simulink library "RFFTLib"  (R2022b)
settings: Solver=VariableStepAuto  StartTime=0.0  StopTime=10.0  RelTol=1e-3
settings Model: Creator=ud1041536  LastModifiedBy=kl13806
settings SolverCC: AlgebraicLoopSolver=TrustRegion
settings DebuggingCC: UnconnectedInputMsg=warning  UnconnectedOutputMsg=warning  UnconnectedLineMsg=warning  SFMachineParentedDataDiag=warning  ArithmeticOperatorsInVariantConditions=warning
settings ModelReferenceCC: EnableRefExpFcnMdlSchedulingChecks=on
settings SFSimCC: CustomCodeUndefinedFunction=UseInterfaceOnly
settings RTWCC: DLArmComputeVersion=19.05

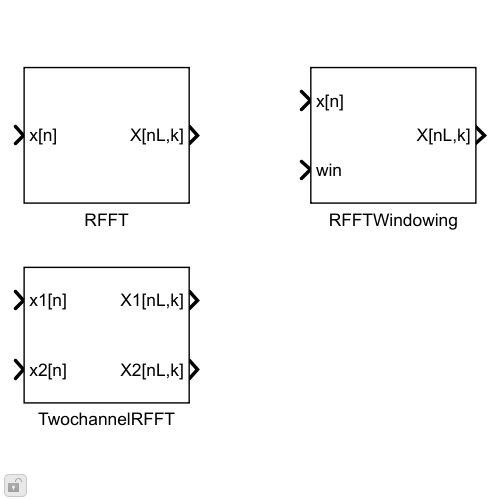
[thumbnail: Simulink's stored preview of the top-level diagram]
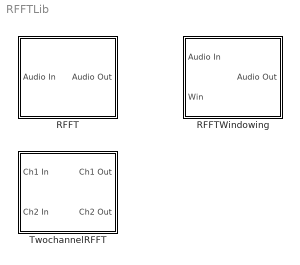
== system RFFTLib ==
  RFFT : Subsystem  mask(Real FFT){variantSelect=Core, fftSize=256, bufferAlias=default}
      mask prompts: variantSelect "Implementation:"; fftSize "FFT size"; bufferAlias "Alias (must be unique across all instances in model)"
      mask help:
      | This block computes the Fourier Transform using an optimized FFT for real inputs. It only supports even number of channels, and 128-point or 256-point FFT.
      |
      | 2 current implementation types are:
      | (i) Core
      | (ii) Generic
      mask init:
      | RfftMaskInit(gcbh, fftSize, bufferAlias, variantSelect)
      mask TypeOptions variantSelect: Core | Generic
      mask Display:
      | port_label('input',1,'x[n]')
      | port_label('output',1,'X[nL,k]')
  RFFTWindowing : Subsystem  mask(Real FFT with In-place Windowing){variantSelect=Core, fftSize=256, bufferAlias=default}
      mask prompts: variantSelect "Implementation:"; fftSize "FFT size"; bufferAlias "Alias (must be unique across all instances in model)"
      mask help:
      | This block performs in-place windowing followed by an optimized FFT computation for real inputs. It only supports even number of channels, and 128-point or 256-point FFT.
      |
      | 2 current implementation types are:
      | (i) Core
      | (ii) Generic
      mask init:
      | RfftMaskInit(gcbh, fftSize, bufferAlias, variantSelect)
      mask TypeOptions variantSelect: Core | Generic
      mask Display:
      | port_label('input',1,'x[n]')
      | port_label('input',2,'win')
      | port_label('output',1,'X[nL,k]')
  TwochannelRFFT : Subsystem  mask(In-place Real FFT){variantSelect=Core, fftSize=256, bufferAlias=default}
      mask prompts: variantSelect "Implementation:"; fftSize "FFT size"; bufferAlias "Alias (must be unique across all instances in model)"
      mask help:
      | This block computes the Fourier Transform using an optimized FFT for real 2-channel input. It only supports 128-point or 256-point FFT.
      |
      | 2 current implementation types are:
      | (i) Core
      | (ii) Generic
      |
      | The inputs MUST be configured correctly for the block to work. Please see 'Help' for more information.
      mask init:
      | Rfft2chanMaskInit(gcbh, fftSize, bufferAlias, variantSelect)
      mask Help:
      | <b>How to configure inputs:</b>
      | 
      | - Signal object class: <b>Blocklib.Signal</b>
      | - Storage class: <b>FFT Buffer</b>
      | - Memory section: <b>FFTMemL1DmWordAlign[fftSize]</b>for the first input signal, and <b>FFTMemL1PmWordAlign[fftSize]</b> for the second
      | 
      | 
      | <b>Why this configuration is needed: </b>
      | 
      | Since the Core implementation makes use of the processor SIMD's capability, the function imposes the following memory restrictions:
      | 1. All buffers (inputs, temp, twiddle) must be allocated in internal memory and not on stack.
      | 2. The inputs must be aligned on an address boundary that is a multiple of the FFT size.
      | 3. The first channel is allocated in a separate memory block from the second channel, i.e. the first one in Data memory and the second in Program memory.
      mask TypeOptions variantSelect: Core | Generic
      mask Display:
      | port_label('input',1,'x1[n]')
      | port_label('input',2,'x2[n]')
      | port_label('output',1,'X1[nL,k]')
      | port_label('output',2,'X2[nL,k]')

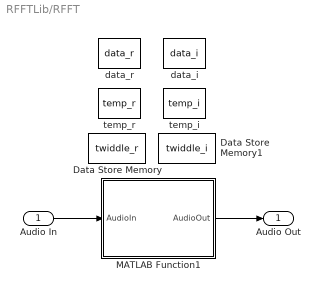
== system RFFTLib/RFFT ==
  Audio In : Inport
  Data Store Memory : DataStoreMemory  DataStoreName=twiddle_r  ReadBeforeWriteMsg=warning  WriteAfterWriteMsg=warning  WriteAfterReadMsg=warning  ShowAdditionalParam=off  OutDataTypeStr=uint32
  Data Store Memory1 : DataStoreMemory  DataStoreName=twiddle_i  ReadBeforeWriteMsg=warning  WriteAfterWriteMsg=warning  WriteAfterReadMsg=warning  ShowAdditionalParam=off  OutDataTypeStr=uint32
  MATLAB Function1 : MATLAB Function  TreatAsAtomicUnit=on
  data_i : DataStoreMemory  DataStoreName=data_i  ReadBeforeWriteMsg=warning  WriteAfterWriteMsg=warning  WriteAfterReadMsg=warning  InitialValue=zeros(fftSize,1)  EmbeddedSignalClassName=Blocklib.Signal  ShowAdditionalParam=off  OutDataTypeStr=single
  data_r : DataStoreMemory  DataStoreName=data_r  ReadBeforeWriteMsg=warning  WriteAfterWriteMsg=warning  WriteAfterReadMsg=warning  InitialValue=zeros(fftSize,1)  EmbeddedSignalClassName=Blocklib.Signal  ShowAdditionalParam=off  OutDataTypeStr=single
  temp_i : DataStoreMemory  DataStoreName=temp_i  ReadBeforeWriteMsg=warning  WriteAfterWriteMsg=warning  WriteAfterReadMsg=warning  InitialValue=zeros(fftSize,1)  EmbeddedSignalClassName=Blocklib.Signal  ShowAdditionalParam=off  OutDataTypeStr=single
  temp_r : DataStoreMemory  DataStoreName=temp_r  ReadBeforeWriteMsg=warning  WriteAfterWriteMsg=warning  WriteAfterReadMsg=warning  InitialValue=zeros(fftSize,1)  EmbeddedSignalClassName=Blocklib.Signal  ShowAdditionalParam=off  OutDataTypeStr=single
  Audio Out : Outport  VectorParamsAs1DForOutWhenUnconnected=off
  wires:
  MATLAB Function1/1(AudioOut) -> Audio Out/1
  Audio In/1 -> MATLAB Function1/1(AudioIn)

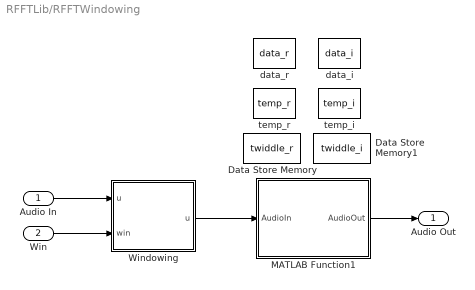
== system RFFTLib/RFFTWindowing ==
  Audio In : Inport
  Win : Inport  Port=2
  Data Store Memory : DataStoreMemory  DataStoreName=twiddle_r  ReadBeforeWriteMsg=warning  WriteAfterWriteMsg=warning  WriteAfterReadMsg=warning  ShowAdditionalParam=off  OutDataTypeStr=uint32
  Data Store Memory1 : DataStoreMemory  DataStoreName=twiddle_i  ReadBeforeWriteMsg=warning  WriteAfterWriteMsg=warning  WriteAfterReadMsg=warning  ShowAdditionalParam=off  OutDataTypeStr=uint32
  MATLAB Function1 : MATLAB Function  TreatAsAtomicUnit=on
  Windowing : MATLAB Function  TreatAsAtomicUnit=on
  data_i : DataStoreMemory  DataStoreName=data_i  ReadBeforeWriteMsg=warning  WriteAfterWriteMsg=warning  WriteAfterReadMsg=warning  InitialValue=zeros(fftSize,1)  EmbeddedSignalClassName=Blocklib.Signal  ShowAdditionalParam=off  OutDataTypeStr=single
  data_r : DataStoreMemory  DataStoreName=data_r  ReadBeforeWriteMsg=warning  WriteAfterWriteMsg=warning  WriteAfterReadMsg=warning  InitialValue=zeros(fftSize,1)  EmbeddedSignalClassName=Blocklib.Signal  ShowAdditionalParam=off  OutDataTypeStr=single
  temp_i : DataStoreMemory  DataStoreName=temp_i  ReadBeforeWriteMsg=warning  WriteAfterWriteMsg=warning  WriteAfterReadMsg=warning  InitialValue=zeros(fftSize,1)  EmbeddedSignalClassName=Blocklib.Signal  ShowAdditionalParam=off  OutDataTypeStr=single
  temp_r : DataStoreMemory  DataStoreName=temp_r  ReadBeforeWriteMsg=warning  WriteAfterWriteMsg=warning  WriteAfterReadMsg=warning  InitialValue=zeros(fftSize,1)  EmbeddedSignalClassName=Blocklib.Signal  ShowAdditionalParam=off  OutDataTypeStr=single
  Audio Out : Outport  VectorParamsAs1DForOutWhenUnconnected=off
  wires:
  MATLAB Function1/1(AudioOut) -> Audio Out/1
  Windowing/1(u) -> MATLAB Function1/1(AudioIn)
  Win/1 -> Windowing/2(win)
  Audio In/1 -> Windowing/1("u ")

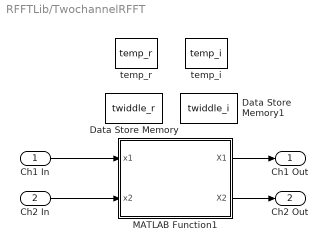
== system RFFTLib/TwochannelRFFT ==
  Ch1 In : Inport
  Ch2 In : Inport  Port=2
  Data Store Memory : DataStoreMemory  DataStoreName=twiddle_r  ReadBeforeWriteMsg=warning  WriteAfterWriteMsg=warning  WriteAfterReadMsg=warning  ShowAdditionalParam=off  OutDataTypeStr=uint32
  Data Store Memory1 : DataStoreMemory  DataStoreName=twiddle_i  ReadBeforeWriteMsg=warning  WriteAfterWriteMsg=warning  WriteAfterReadMsg=warning  ShowAdditionalParam=off  OutDataTypeStr=uint32
  MATLAB Function1 : MATLAB Function  TreatAsAtomicUnit=on
  temp_i : DataStoreMemory  DataStoreName=temp_i  ReadBeforeWriteMsg=warning  WriteAfterWriteMsg=warning  WriteAfterReadMsg=warning  InitialValue=zeros(fftSize,1)  EmbeddedSignalClassName=Blocklib.Signal  ShowAdditionalParam=off  OutDataTypeStr=single
  temp_r : DataStoreMemory  DataStoreName=temp_r  ReadBeforeWriteMsg=warning  WriteAfterWriteMsg=warning  WriteAfterReadMsg=warning  InitialValue=zeros(fftSize,1)  EmbeddedSignalClassName=Blocklib.Signal  ShowAdditionalParam=off  OutDataTypeStr=single
  Ch1 Out : Outport  VectorParamsAs1DForOutWhenUnconnected=off
  Ch2 Out : Outport  Port=2  VectorParamsAs1DForOutWhenUnconnected=off
  wires:
  MATLAB Function1/1(X1) -> Ch1 Out/1
  Ch1 In/1 -> MATLAB Function1/1(x1)
  Ch2 In/1 -> MATLAB Function1/2(x2)
  MATLAB Function1/2(X2) -> Ch2 Out/1

== matlab function RFFTLib/RFFT/MATLAB Function1 ==
  data: AudioIn input; AudioOut output; fftSize parameter; temp_r data_store_memory; temp_i data_store_memory; data_r data_store_memory; data_i data_store_memory; twiddle_r data_store_memory; twiddle_i data_store_memory; variantSelect parameter
function AudioOut = fftReal(AudioIn, fftSize, variantSelect)   

global data_r
global data_i
global temp_r
global temp_i
global twiddle_r
global twiddle_i

[~, numChannels] = size(AudioIn);
spectrumSize = (fftSize/2) + 1;

% Nullcopy copies type, size, and complexity of input to output
AudioOut = coder.nullcopy(complex(single(zeros(spectrumSize, numChannels))));

% Set correct data types
fftSize = uint32(fftSize);
numChannels = uint32(numChannels);

% There are two implementation types:
% Type    Value   Description
% CORE    1       Optimized assembly running on SHARC+ core
% GENERIC 2       Generic implementation for other targets without CRL

% Simulation
if(coder.target('MATLAB') || coder.target('Sfun')) 
    AudioOut = rfft_simulation(AudioIn, fftSize); 
    
% Code generation
else
    % Core
    if (variantSelect == 1) 
        % Set the twiddle pointers to correct twiddle table
        % The pointers are of type uint32 here and will be casted to float* 
        % in the code-replaced function. The twiddle tables are declared in 
        % a separate file and will be pulled in through CRL.
        if fftSize == 256
            coder.ceval('set_twiddle_256', coder.wref(twiddle_r), coder.wref(twiddle_i));
        else
            coder.ceval('set_twiddle_128', coder.wref(twiddle_r), coder.wref(twiddle_i));
        end
        AudioOut = rfft_process(AudioIn, data_r, data_i, temp_r, temp_i, ...
            twiddle_r, twiddle_i, fftSize, numChannels);
        
    % Generic
    else
        AudioOut = rfft_simulation(AudioIn, fftSize);       
    end
end

end

%% CRL function for code generation
function y = rfft_process(u, data_r, data_i, temp_r, temp_i, ...
    twiddle_r, twiddle_i, fft_size, num_channels)
% If target == codegen, error out if no CRL found
coder.replace('-errorifnoreplacement');
y = complex(single(zeros((fft_size/2) + 1, num_channels)));

end

%% Function for simulation
function y = rfft_simulation(u, fft_size)

half_spectrum_size = (fft_size/2) + 1;
y = fft(u); 
y = y(1:half_spectrum_size, :); % get half spectrum

end

== matlab function RFFTLib/RFFTWindowing/MATLAB Function1 ==
  data: AudioIn input; AudioOut output; fftSize parameter; temp_r data_store_memory; temp_i data_store_memory; data_r data_store_memory; data_i data_store_memory; twiddle_r data_store_memory; twiddle_i data_store_memory; variantSelect parameter
function AudioOut = fftReal(AudioIn, fftSize, variantSelect)   

global data_r
global data_i
global temp_r
global temp_i
global twiddle_r
global twiddle_i

[~, numChannels] = size(AudioIn);
spectrumSize = (fftSize/2) + 1;

% Nullcopy copies type, size, and complexity of input to output
AudioOut = coder.nullcopy(complex(single(zeros(spectrumSize, numChannels))));

% Set correct data types
fftSize = uint32(fftSize);
numChannels = uint32(numChannels);

% There are two implementation types:
% Type    Value   Description
% CORE    1       Optimized assembly running on SHARC+ core
% GENERIC 2       Generic implementation for other targets without CRL

% Simulation
if(coder.target('MATLAB') || coder.target('Sfun')) 
    AudioOut = rfft_simulation(AudioIn, fftSize); 
    
% Code generation
else
    % Core
    if (variantSelect == 1) 
        % Set the twiddle pointers to correct twiddle table
        % The pointers are of type uint32 here and will be casted to float* 
        % in the code-replaced function. The twiddle tables are declared in 
        % a separate file and will be pulled in through CRL.
        if fftSize == 256
            coder.ceval('set_twiddle_256', coder.wref(twiddle_r), coder.wref(twiddle_i));
        else
            coder.ceval('set_twiddle_128', coder.wref(twiddle_r), coder.wref(twiddle_i));
        end
        AudioOut = rfft_process(AudioIn, data_r, data_i, temp_r, temp_i, ...
            twiddle_r, twiddle_i, fftSize, numChannels);
        
    % Generic
    else
        AudioOut = rfft_simulation(AudioIn, fftSize);       
    end
end

end

%% CRL function for code generation
function y = rfft_process(u, data_r, data_i, temp_r, temp_i, ...
    twiddle_r, twiddle_i, fft_size, num_channels)
% If target == codegen, error out if no CRL found
coder.replace('-errorifnoreplacement');
y = complex(single(zeros((fft_size/2) + 1, num_channels)));

end

%% Function for simulation
function y = rfft_simulation(u, fft_size)

half_spectrum_size = (fft_size/2) + 1;
y = fft(u); 
y = y(1:half_spectrum_size, :); % get half spectrum

end

== matlab function RFFTLib/TwochannelRFFT/MATLAB Function1 ==
  data: x1 input; x2 input; X1 output; fftSize parameter; temp_r data_store_memory; temp_i data_store_memory; X2 output; twiddle_r data_store_memory; twiddle_i data_store_memory; variantSelect parameter
function [X1, X2] = fftReal(x1, x2, fftSize, variantSelect)   

global temp_r
global temp_i
global twiddle_r
global twiddle_i

% Nullcopy copies type, size, and complexity to output
X1 = coder.nullcopy(complex(single(zeros((fftSize/2) + 1, 1))));
X2 = coder.nullcopy(complex(single(zeros((fftSize/2) + 1, 1))));

% Set correct data types
fftSize = uint32(fftSize);

% There are two implementation types:
% Type    Value   Description
% CORE    1       Optimized assembly running on SHARC+ core
% GENERIC 2       Generic implementation for other targets without CRL

% Simulation
if(coder.target('MATLAB') || coder.target('Sfun')) 
    [X1, X2] = rfft_inplace_simulation(x1, x2, fftSize);

% Code generation
else
    % Core
    if (variantSelect == 1) 
        % Set the twiddle pointers to correct twiddle table
        % The pointers are of type uint32 here and will be casted to float* 
        % in the code-replaced function. The twiddle tables are declared in 
        % a separate file and will be pulled in through CRL.
        if fftSize == 256
            coder.ceval('set_twiddle_256', coder.wref(twiddle_r), coder.wref(twiddle_i));
        else
            coder.ceval('set_twiddle_128', coder.wref(twiddle_r), coder.wref(twiddle_i));
        end
        [X1, X2] = rfft_inplace_process(x1, x2, temp_r, temp_i, ...
            twiddle_r, twiddle_i, fftSize);
    
    % Generic
    else
        [X1, X2] = rfft_inplace_simulation(x1, x2, fftSize);
    end
end
    
end

%% CRL function for code generation
function [y1, y2] = rfft_inplace_process(u1, u2, temp_r, temp_i, ...
    twiddle_r, twiddle_i, fft_size)
% If target == codegen, error out if no CRL found
coder.replace('-errorifnoreplacement');

half_spectrum_size = (fft_size/2) + 1;
y1 = complex(single(zeros(half_spectrum_size, 1)));
y2 = complex(single(zeros(half_spectrum_size, 1)));

end

%% Function for simulation
function [y1, y2] = rfft_inplace_simulation(u1, u2, fft_size)

half_spectrum_size = (fft_size/2) + 1;
x = complex(single(zeros(fft_size, 2)));
y1 = complex(single(zeros(half_spectrum_size, 1)));
y2 = complex(single(zeros(half_spectrum_size, 1)));

% compute FFT
x(:,1) = fft(u1);
x(:,2) = fft(u2);

% get half spectrum
y1 = x(1:half_spectrum_size, 1);
y2 = x(1:half_spectrum_size, 2);

end

== matlab function RFFTLib/RFFTWindowing/Windowing ==
  data: u input; win input; u output
function u = fcn(u, win)

% Get sizes
[~, numChannels] = size(u);

% Loop since array-vector multiply operation doesn't work here
% Input/Output have the same variable name for in-place processing
for i = 1:numChannels
    u(:, i) = u(:,i) .* win;
end

end
